simulink model "TrqArb"  (R2023a)
settings: Solver=FixedStepDiscrete  StartTime=0.0  StopTime=10  FixedStep=0.01  RelTol=1e-3
model workspace (MAT data in the model file):
  Cal_TrqMax = Simulink.Parameter
  Cal_TrqMax.Value = 1500
  Cal_TrqMax.DataType = 'single'
  Cal_TrqMax.Min = 0
  Cal_TrqMax.Max = 2000
  Cal_TrqMax.Complexity = 'real'
  Cal_TrqMax.Dimensions = [1 1]
  Cal_TrqRate = Simulink.Parameter
  Cal_TrqRate.Value = 2000
  Cal_TrqRate.DataType = 'single'
  Cal_TrqRate.Min = 0
  Cal_TrqRate.Max = 5000
  Cal_TrqRate.Complexity = 'real'
  Cal_TrqRate.Dimensions = [1 1]
settings Model: Creator=Henry  LastModifiedBy=Henry
settings OptimizationCC: DefaultParameterBehavior=Inlined  EnhancedBackFolding=on  PassReuseOutputArgsAs=Individual arguments  ZeroExternalMemoryAtStartup=off  OptimizeBlockOrder=speed  DifferentSizesBufferReuse=on  OptimizationCustomize=off  EfficientTunableParamExpr=on
settings DebuggingCC: ParameterTunabilityLossMsg=error
settings SFSimCC: MATLABDynamicMemAlloc=off
settings RTWCC: Description=AUTOSAR  SystemTargetFile=autosar.tlc  GenCodeOnly=on  TemplateMakefile=ert_default_tmf  GenerateReport=on
settings CodeAppCC: ForceParamTrailComments=on  IgnoreCustomStorageClasses=off  OperatorAnnotations=on  SimulinkDataObjDesc=on  SFDataObjDesc=on  InsertBlockDesc=on
settings STFCustomTargetCC: MultiwordLength=256  ParMdlRefBuildCompliant=on  CompOptLevelCompliant=on  ConcurrentExecutionCompliant=off  IncludeMdlTerminateFcn=off  CombineOutputUpdateFcns=on  SuppressErrorStatus=on  ERTCustomFileBanners=on  CodeInterfacePackaging=Reusable function  SupportNonFinite=off  SupportComplex=off  SupportContinuousTime=off  SupportNonInlinedSFcns=off  RemoveResetFunc=on  MATLABClassNameForMDSCustomization=Simulink.SoftwareTarget.ERTCustomization  AutosarCompliant=on  GRTInterface=off  LookupTableObjectStructAxisOrder=2,1,3,4,...  LUTObjectStructOrderEvenSpacing=Size,Table,Breakpoints  SystemTargetFile=autosar.tlc
settings ERTTargetCC: TargetLangStandard=C99 (ISO)  ConcurrentExecutionCompliant=off  IncludeMdlTerminateFcn=off  SuppressErrorStatus=on  CodeInterfacePackaging=Reusable function  SupportNonFinite=off  SupportComplex=off  ModelStepFunctionPrototypeControlCompliant=off  CPPClassGenCompliant=off  AutosarCompliant=on  LookupTableObjectStructAxisOrder=2,1,3,4,...  LUTObjectStructOrderEvenSpacing=Size,Table,Breakpoints  InlinedParameterPlacement=NonHierarchical  ERTCustomFileTemplate=example_file_process.tlc

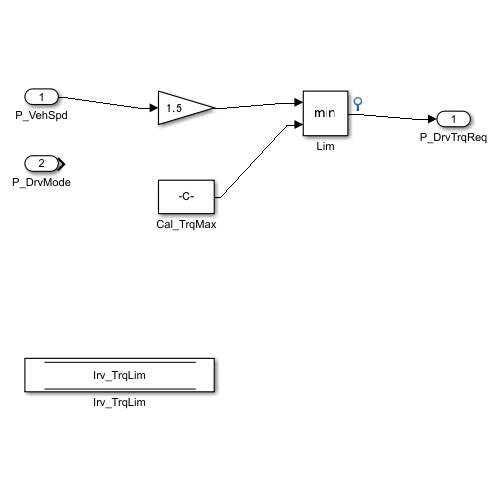
[thumbnail: Simulink's stored preview of the top-level diagram]
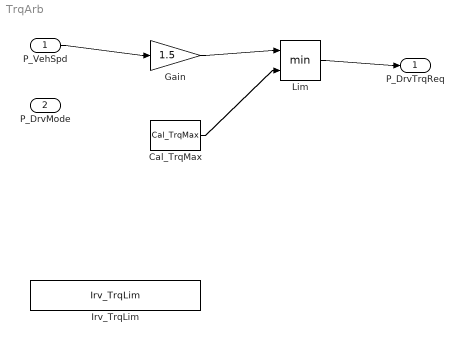
== system TrqArb ==
  P_VehSpd : Inport  OutDataTypeStr=single
  P_DrvMode : Inport  Port=2  OutDataTypeStr=Enum: En_DrvMode
  Cal_TrqMax : Constant  Value=Cal_TrqMax  OutDataTypeStr=single
  Gain : Gain  Gain=1.5  OutDataTypeStr=single
  Irv_TrqLim : DataStoreMemory  DataStoreName=Irv_TrqLim  WriteAfterWriteMsg=warning  ShowAdditionalParam=off  OutDataTypeStr=single
  Lim : MinMax  Inputs=2  OutDataTypeStr=single
  P_DrvTrqReq : Outport  OutDataTypeStr=single
  wires:
  P_VehSpd/1 -> Gain/1
  Gain/1 -> Lim/1
  Cal_TrqMax/1 -> Lim/2
  Lim/1 -> P_DrvTrqReq/1
